simulink model "NeuralNetwork"  (R2016a)
settings: Solver=VariableStepAuto  StartTime=0.0  StopTime=100  RelTol=1e-3
values from neighbouring files (symbols this model uses):
  A0 = 0.5e-4    (= 5e-05)    [BPAndPID.m]
  cong = [1,1,1]/3600*d2r    [BPAndPID.m]
  fei1 = [5,5,5]'*d2r    [BPAndPID.m]
  HB0 = [IB*Wwo]'    [BPAndPID.m]
  invIB = inv(IB)    [BPAndPID.m]
  Noig = [1,1,1]*1/3*5*10^(-5)*d2r    [BPAndPID.m]
  Q0 = [Q1 Q2 Q3]    [BPAndPID.m]
  Q00 = 0.6736    [BPAndPID.m]
  Qt = [qt0 qt1 qt2 qt3]    [BPAndPID.m]
  Tscontrol = 0.05    [BPAndPID.m]
  Wc = [0 0 0]    [BPAndPID.m]
  Wio = [0 0.001 0]'    [BPAndPID.m]
libraries: aerolibutil x1
settings Model: Creator=lenovo  LastModifiedBy=lenovo

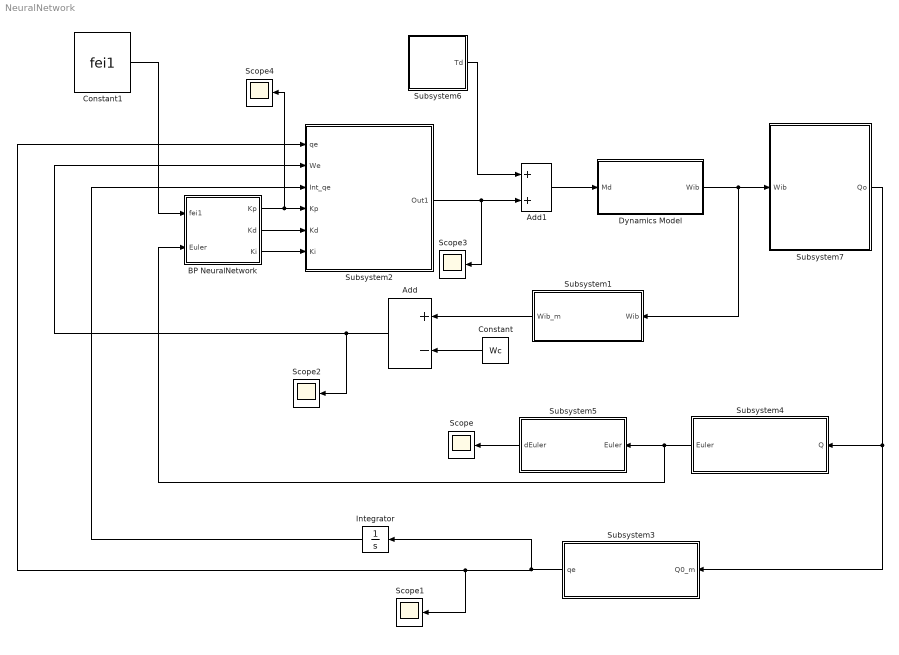
== system NeuralNetwork ==
  Add : Sum  Inputs=+-
  Add1 : Sum
  BP NeuralNetwork : Subsystem
  Constant : Constant  Value=Wc
  Constant1 : Constant  Value=fei1
  Dynamics Model : Subsystem
  Integrator : Integrator
  Scope{,1..4} (5 alike) : Scope
  Subsystem1 : Subsystem
      mask Display:
      | disp('Gyro')
      | port_label('input',1,'Wib')
      | port_label('output',1,'Wib_m')
  Subsystem2 : Subsystem
      mask Display:
      | disp('Controller')
      | port_label('input',1,'qe')
      | port_label('input',2,'we')
      | port_label('input',3,'int_qe')
      | port_label('input',4,'Kp')
      | port_label('input',5,'Kd')
      | port_label('input',6,'Ki')
      | port_label('output',1,'T')
  Subsystem3 : Subsystem
      mask Display:
      | disp('Target')
      | port_label('input',1,'Q')
      | port_label('output',1,'qe')
  Subsystem4 : Subsystem
      mask Display:
      | disp('Quaternion2Euler')
      | port_label('input',1,'Q')
      | port_label('output',1,'Euler')
  Subsystem5 : Subsystem
      mask Display:
      | disp('EulerError')
      | port_label('input',1,'Euler')
      | port_label('output',1,'dEuler')
  Subsystem6 : Subsystem
  Subsystem7 : Subsystem
      mask Display:
      | disp('Kinematics')
      | port_label('input',1,'Wib')
      | port_label('output',1,'Q')
  wires:
  Dynamics Model/1(Wib) -> Subsystem1/1(Wib), Subsystem7/1(Wib)
  Subsystem3/1(qe) -> Scope1/1, Subsystem2/1(qe), Integrator/1
  Subsystem7/1(Qo) -> Subsystem3/1(Q0_m), Subsystem4/1(Q)
  Subsystem5/1(dEuler) -> Scope/1
  Subsystem1/1(Wib_m) -> Add/1
  Constant/1 -> Add/2
  Add/1 -> Scope2/1, Subsystem2/2(We)
  Add1/1 -> Dynamics Model/1(Md)
  Subsystem2/1(Out1) -> Scope3/1, Add1/2
  Subsystem6/1(Td) -> Add1/1
  Integrator/1 -> Subsystem2/3(Int_qe)
  BP NeuralNetwork/1(Kp) -> Scope4/1, Subsystem2/4(Kp)
  BP NeuralNetwork/2(Kd) -> Subsystem2/5(Kd)
  BP NeuralNetwork/3(Ki) -> Subsystem2/6(Ki)
  Constant1/1 -> BP NeuralNetwork/1(fei1)
  Subsystem4/1(Euler) -> BP NeuralNetwork/2(Euler), Subsystem5/1(Euler)

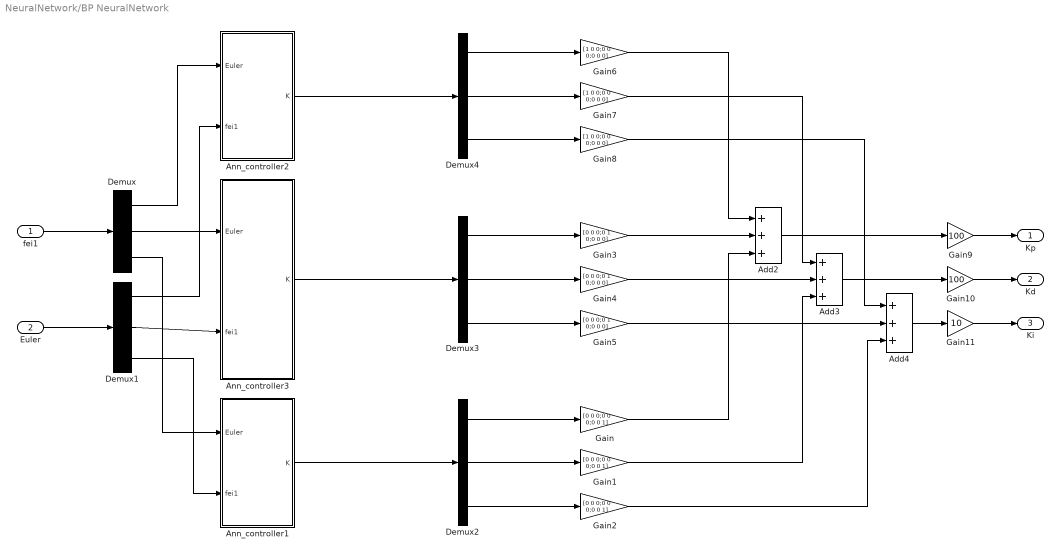
== system NeuralNetwork/BP NeuralNetwork ==
  fei1 : Inport
  Euler : Inport  Port=2
  Add2 : Sum  Inputs=+++
  Add3 : Sum  Inputs=+++
  Add4 : Sum  Inputs=+++
  Ann_controller1 : Subsystem
  Ann_controller2 : Subsystem
  Ann_controller3 : Subsystem
  Demux{,2..4} (4 alike) : Demux  Outputs=[1 1 1]
  Demux1 : Demux  Outputs=[1;1;1]
  Gain : Gain  Gain=[0 0 0;0 0 0;0 0 1]
  Gain1 : Gain  Gain=[0 0 0;0 0 0;0 0 1]
  Gain10 : Gain  Gain=100
  Gain11 : Gain  Gain=10
  Gain2 : Gain  Gain=[0 0 0;0 0 0;0 0 1]
  Gain3 : Gain  Gain=[0 0 0;0 1 0;0 0 0]
  Gain4 : Gain  Gain=[0 0 0;0 1 0;0 0 0]
  Gain5 : Gain  Gain=[0 0 0;0 1 0;0 0 0]
  Gain6 : Gain  Gain=[1 0 0;0 0 0;0 0 0]
  Gain7 : Gain  Gain=[1 0 0;0 0 0;0 0 0]
  Gain8 : Gain  Gain=[1 0 0;0 0 0;0 0 0]
  Gain9 : Gain  Gain=100
  Kp : Outport
  Kd : Outport  Port=2
  Ki : Outport  Port=3
  wires:
  Gain2/1 -> Add4/3
  Demux4/2 -> Gain7/1
  Demux2/3 -> Gain2/1
  Demux3/1 -> Gain3/1
  Gain6/1 -> Add2/1
  Gain3/1 -> Add2/2
  Demux2/2 -> Gain1/1
  Demux1/3 -> Ann_controller1/2(fei1)
  Demux3/2 -> Gain4/1
  Demux/1 -> Ann_controller2/1(Euler)
  Gain5/1 -> Add4/2
  Demux3/3 -> Gain5/1
  Demux2/1 -> Gain/1
  Demux4/3 -> Gain8/1
  Ann_controller2/1(K) -> Demux4/1
  Demux4/1 -> Gain6/1
  Gain/1 -> Add2/3
  Gain4/1 -> Add3/2
  Gain7/1 -> Add3/1
  Gain1/1 -> Add3/3
  Demux1/2 -> Ann_controller3/2(fei1)
  Demux1/1 -> Ann_controller2/2(fei1)
  Ann_controller3/1(K) -> Demux3/1
  Ann_controller1/1(K) -> Demux2/1
  Gain8/1 -> Add4/1
  Demux/2 -> Ann_controller3/1(Euler)
  fei1/1 -> Demux/1
  Euler/1 -> Demux1/1
  Add3/1 -> Gain10/1
  Add4/1 -> Gain11/1
  Add2/1 -> Gain9/1
  Gain9/1 -> Kp/1
  Gain10/1 -> Kd/1
  Gain11/1 -> Ki/1
  Demux/3 -> Ann_controller1/1(Euler)

== system NeuralNetwork/Dynamics Model ==
  note: W X H
  note: W
  note: H
  note: dH
  Md : Inport
  Add : Sum  Inputs=-+
  Gain : Gain  Gain=invIB  Multiplication=Matrix(u*K)
  Gain1 : Gain  Gain=-1
  Integrator : Integrator  InitialCondition=HB0
  Subsystem : Subsystem
      mask Display:
      | disp('Cross \nProduct')
      | port_label('input',1,'X')
      | port_label('input',2,'Y')
      | port_label('output',1,'X*Y')
  Wib : Outport
  wires:
  Integrator/1 -> Gain/1, Subsystem/2(Y)
  Gain/1 -> Wib/1, Gain1/1
  Add/1 -> Integrator/1
  Md/1 -> Add/2
  Gain1/1 -> Subsystem/1(X)
  Subsystem/1(X*Y) -> Add/1

== system NeuralNetwork/Subsystem1 ==
  Wib : Inport
  Add : Sum  Inputs=+++
  ConstantDrifting : Constant  Value=cong
  Gain : Gain  Gain=Noig
  Quantizer : Quantizer  QuantizationInterval=Gyquan
  WhiteNoise : RandomNumber  Mean=[0,0,0]  Variance=[1,1,1]  Seed=fix(abs(10000*rand([3,1])))  SampleTime=Tscontrol
  Wib_m : Outport
  wires:
  Quantizer/1 -> Wib_m/1
  Wib/1 -> Add/2
  Add/1 -> Quantizer/1
  ConstantDrifting/1 -> Add/3
  Gain/1 -> Add/1
  WhiteNoise/1 -> Gain/1

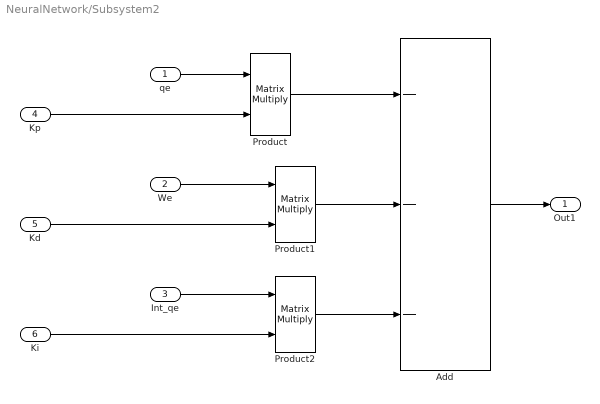
== system NeuralNetwork/Subsystem2 ==
  qe : Inport
  We : Inport  Port=2
  Int_qe : Inport  Port=3
  Kp : Inport  Port=4
  Kd : Inport  Port=5
  Ki : Inport  Port=6
  Add : Sum  Inputs=---
  Product : Product  Multiplication=Matrix(*)
  Product1 : Product  Multiplication=Matrix(*)
  Product2 : Product  Multiplication=Matrix(*)
  Out1 : Outport
  wires:
  Add/1 -> Out1/1
  Product/1 -> Add/1
  Kd/1 -> Product1/2
  We/1 -> Product1/1
  Product1/1 -> Add/2
  Kp/1 -> Product/2
  qe/1 -> Product/1
  Product2/1 -> Add/3
  Ki/1 -> Product2/2
  Int_qe/1 -> Product2/1

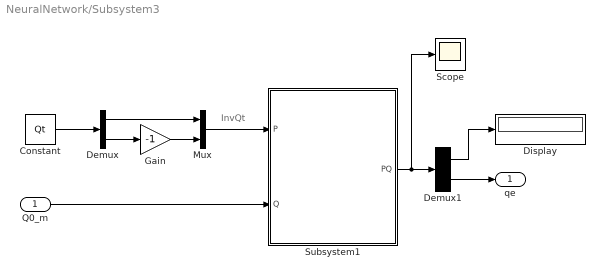
== system NeuralNetwork/Subsystem3 ==
  note: InvQt
  Q0_m : Inport
  Constant : Constant  Value=Qt
  Demux : Demux  Outputs=2
  Demux1 : Demux  Outputs=[1 3]
  Display : Display
  Gain : Gain  Gain=-1
  Mux : Mux  Inputs=2
  Scope : Scope
  Subsystem1 : Subsystem
      mask Display:
      | disp('InterQ Multiply')
      | port_label('input',1,'P')
      | port_label('input',2,'Q')
      | port_label('output',1,'PQ')
  qe : Outport
  wires:
  Subsystem1/1(PQ) -> Scope/1, Demux1/1
  Constant/1 -> Demux/1
  Demux/1 -> Mux/1
  Demux/2 -> Gain/1
  Gain/1 -> Mux/2
  Q0_m/1 -> Subsystem1/2(Q)
  Mux/1 -> Subsystem1/1(P)
  Demux1/2 -> qe/1
  Demux1/1 -> Display/1

== system NeuralNetwork/Subsystem4 ==
  Q : Inport
  Mux : Mux  Inputs=3
  Phi : Fcn  Expr=atan(2*(u(1)*u(4)-u(3)*u(2))/(2*(u(1)^2+u(3)^2)-1))
  Psi : Fcn  Expr=atan(2*(u(1)*u(3)-u(2)*u(4))/(2*(u(1)^2+u(4)^2)-1))
  Scope : Scope
  Theta : Fcn  Expr=asin(2*(u(1)*u(2)+u(4)*u(3)))
  Euler : Outport
  wires:
  Mux/1 -> Scope/1, Euler/1
  Q/1 -> Theta/1, Phi/1, Psi/1
  Theta/1 -> Mux/3
  Psi/1 -> Mux/1
  Phi/1 -> Mux/2

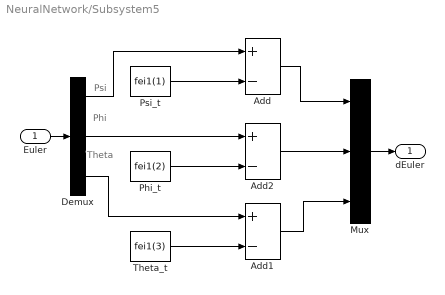
== system NeuralNetwork/Subsystem5 ==
  note: Psi
  note: Theta
  note: Phi
  Euler : Inport
  Add : Sum  Inputs=+-
  Add1 : Sum  Inputs=+-
  Add2 : Sum  Inputs=+-
  Demux : Demux  Outputs=[1 1 1]
  Mux : Mux  Inputs=3
  Phi_t : Constant  Value=fei1(2)
  Psi_t : Constant  Value=fei1(1)
  Theta_t : Constant  Value=fei1(3)
  dEuler : Outport
  wires:
  Demux/1 -> Add/1
  Mux/1 -> dEuler/1
  Euler/1 -> Demux/1
  Theta_t/1 -> Add1/2
  Add/1 -> Mux/1
  Demux/3 -> Add1/1
  Add2/1 -> Mux/2
  Psi_t/1 -> Add/2
  Demux/2 -> Add2/1
  Phi_t/1 -> Add2/2
  Add1/1 -> Mux/3

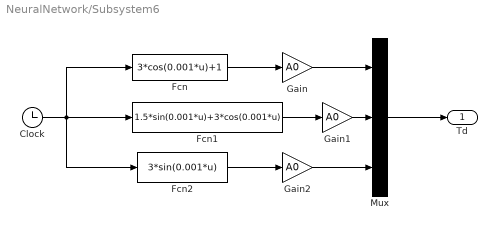
== system NeuralNetwork/Subsystem6 ==
  Clock : Clock
  Fcn : Fcn  Expr=3*cos(0.001*u)+1
  Fcn1 : Fcn  Expr=1.5*sin(0.001*u)+3*cos(0.001*u)
  Fcn2 : Fcn  Expr=3*sin(0.001*u)
  Gain : Gain  Gain=A0
  Gain1 : Gain  Gain=A0
  Gain2 : Gain  Gain=A0
  Mux : Mux  Inputs=3
  Td : Outport
  wires:
  Gain/1 -> Mux/1
  Mux/1 -> Td/1
  Clock/1 -> Fcn2/1, Fcn/1, Fcn1/1
  Fcn2/1 -> Gain2/1
  Fcn1/1 -> Gain1/1
  Fcn/1 -> Gain/1
  Gain2/1 -> Mux/3
  Gain1/1 -> Mux/2

== system NeuralNetwork/Subsystem7 ==
  Wib : Inport
  Add1 : Sum  Inputs=+-
  Constant : Constant  Value=Wio
  Product1 : Product  Multiplication=Matrix(*)
  Subsystem1 : Subsystem
      mask Display:
      | disp('Quaternion2 \nAttitudeMarix')
      | port_label('input',1,'Qua')
      | port_label('output',1,'Marix')
  Subsystem5 : Subsystem
      mask Display:
      | disp('Quaternion \nSolve Model')
      | port_label('input',1,'Wob')
      | port_label('output',1,'Qo')
  Qo : Outport
  wires:
  Subsystem5/1(Out1) -> Qo/1, Subsystem1/1(Quaternion)
  Constant/1 -> Product1/2
  Subsystem1/1("AttitudeMarix ") -> Product1/1
  Add1/1 -> Subsystem5/1(In1)
  Wib/1 -> Add1/1
  Product1/1 -> Add1/2

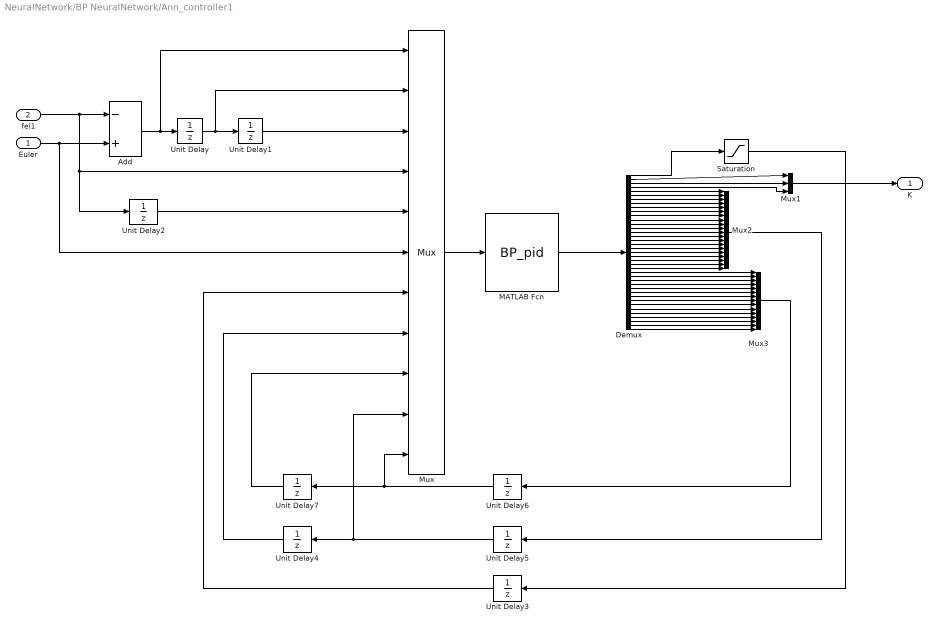
== system NeuralNetwork/BP NeuralNetwork/Ann_controller1 ==
  Euler : Inport
  fei1 : Inport  Port=2
  Add : Sum  Inputs=-+
  Demux : Demux  Outputs=39
  MATLAB Fcn : MATLABFcn  MATLABFcn=BP_pid  Output1D=off
  Mux : Mux  Inputs=11
  Mux1 : Mux  Inputs=3
  Mux2 : Mux  Inputs=20
  Mux3 : Mux  Inputs=15
  Saturation : Saturate  UpperLimit=1  LowerLimit=0
  Unit Delay{,1..3} (4 alike) : UnitDelay
  Unit Delay4 : UnitDelay  InitialCondition=rand(20,1)
  Unit Delay5 : UnitDelay  InitialCondition=rand(20,1)
  Unit Delay6 : UnitDelay  InitialCondition=rand(15,1)
  Unit Delay7 : UnitDelay  InitialCondition=rand(15,1)
  K : Outport
  wires:
  Euler/1 -> Mux/6, Add/2
  Add/1 -> Mux/1, Unit Delay/1
  Unit Delay/1 -> Mux/2, Unit Delay1/1
  MATLAB Fcn/1 -> Demux/1
  Unit Delay5/1 -> Unit Delay4/1, Mux/10
  Unit Delay3/1 -> Mux/7
  Unit Delay6/1 -> Unit Delay7/1, Mux/11
  Demux/2 -> Mux1/1
  Demux/3 -> Mux1/2
  Demux/4 -> Mux1/3
  Mux1/1 -> K/1
  Demux/5 -> Mux2/1
  Demux/6 -> Mux2/2
  Demux/7 -> Mux2/3
  Demux/8 -> Mux2/4
  Demux/9 -> Mux2/5
  Demux/10 -> Mux2/6
  Demux/11 -> Mux2/7
  Demux/12 -> Mux2/8
  Demux/13 -> Mux2/9
  Demux/14 -> Mux2/10
  Demux/15 -> Mux2/11
  Demux/16 -> Mux2/12
  Demux/17 -> Mux2/13
  Demux/18 -> Mux2/14
  Demux/19 -> Mux2/15
  Demux/20 -> Mux2/16
  Demux/21 -> Mux2/17
  Demux/22 -> Mux2/18
  Demux/23 -> Mux2/19
  Demux/24 -> Mux2/20
  Mux2/1 -> Unit Delay5/1
  Demux/25 -> Mux3/1
  Demux/26 -> Mux3/2
  Demux/27 -> Mux3/3
  Demux/28 -> Mux3/4
  Demux/29 -> Mux3/5
  Demux/30 -> Mux3/6
  Demux/31 -> Mux3/7
  Demux/32 -> Mux3/8
  Demux/33 -> Mux3/9
  Demux/34 -> Mux3/10
  Demux/35 -> Mux3/11
  Demux/36 -> Mux3/12
  Demux/37 -> Mux3/13
  Demux/38 -> Mux3/14
  Demux/39 -> Mux3/15
  Mux3/1 -> Unit Delay6/1
  Demux/1 -> Saturation/1
  Saturation/1 -> Unit Delay3/1
  Mux/1 -> MATLAB Fcn/1
  Unit Delay7/1 -> Mux/9
  Unit Delay4/1 -> Mux/8
  fei1/1 -> Unit Delay2/1, Mux/4, Add/1
  Unit Delay2/1 -> Mux/5
  Unit Delay1/1 -> Mux/3

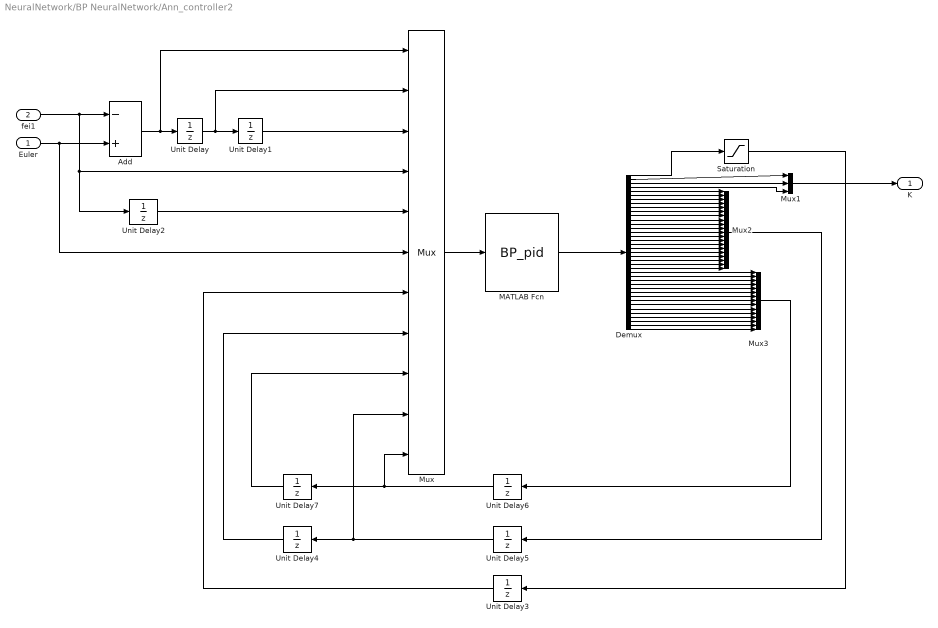
== system NeuralNetwork/BP NeuralNetwork/Ann_controller2 ==
  Euler : Inport
  fei1 : Inport  Port=2
  Add : Sum  Inputs=-+
  Demux : Demux  Outputs=39
  MATLAB Fcn : MATLABFcn  MATLABFcn=BP_pid  Output1D=off
  Mux : Mux  Inputs=11
  Mux1 : Mux  Inputs=3
  Mux2 : Mux  Inputs=20
  Mux3 : Mux  Inputs=15
  Saturation : Saturate  UpperLimit=1  LowerLimit=0
  Unit Delay{,1..3} (4 alike) : UnitDelay
  Unit Delay4 : UnitDelay  InitialCondition=rand(20,1)
  Unit Delay5 : UnitDelay  InitialCondition=rand(20,1)
  Unit Delay6 : UnitDelay  InitialCondition=rand(15,1)
  Unit Delay7 : UnitDelay  InitialCondition=rand(15,1)
  K : Outport
  wires:
  Euler/1 -> Mux/6, Add/2
  Add/1 -> Mux/1, Unit Delay/1
  Unit Delay/1 -> Mux/2, Unit Delay1/1
  MATLAB Fcn/1 -> Demux/1
  Unit Delay5/1 -> Unit Delay4/1, Mux/10
  Unit Delay3/1 -> Mux/7
  Unit Delay6/1 -> Unit Delay7/1, Mux/11
  Demux/2 -> Mux1/1
  Demux/3 -> Mux1/2
  Demux/4 -> Mux1/3
  Mux1/1 -> K/1
  Demux/5 -> Mux2/1
  Demux/6 -> Mux2/2
  Demux/7 -> Mux2/3
  Demux/8 -> Mux2/4
  Demux/9 -> Mux2/5
  Demux/10 -> Mux2/6
  Demux/11 -> Mux2/7
  Demux/12 -> Mux2/8
  Demux/13 -> Mux2/9
  Demux/14 -> Mux2/10
  Demux/15 -> Mux2/11
  Demux/16 -> Mux2/12
  Demux/17 -> Mux2/13
  Demux/18 -> Mux2/14
  Demux/19 -> Mux2/15
  Demux/20 -> Mux2/16
  Demux/21 -> Mux2/17
  Demux/22 -> Mux2/18
  Demux/23 -> Mux2/19
  Demux/24 -> Mux2/20
  Mux2/1 -> Unit Delay5/1
  Demux/25 -> Mux3/1
  Demux/26 -> Mux3/2
  Demux/27 -> Mux3/3
  Demux/28 -> Mux3/4
  Demux/29 -> Mux3/5
  Demux/30 -> Mux3/6
  Demux/31 -> Mux3/7
  Demux/32 -> Mux3/8
  Demux/33 -> Mux3/9
  Demux/34 -> Mux3/10
  Demux/35 -> Mux3/11
  Demux/36 -> Mux3/12
  Demux/37 -> Mux3/13
  Demux/38 -> Mux3/14
  Demux/39 -> Mux3/15
  Mux3/1 -> Unit Delay6/1
  Demux/1 -> Saturation/1
  Saturation/1 -> Unit Delay3/1
  Mux/1 -> MATLAB Fcn/1
  Unit Delay7/1 -> Mux/9
  Unit Delay4/1 -> Mux/8
  fei1/1 -> Unit Delay2/1, Mux/4, Add/1
  Unit Delay2/1 -> Mux/5
  Unit Delay1/1 -> Mux/3

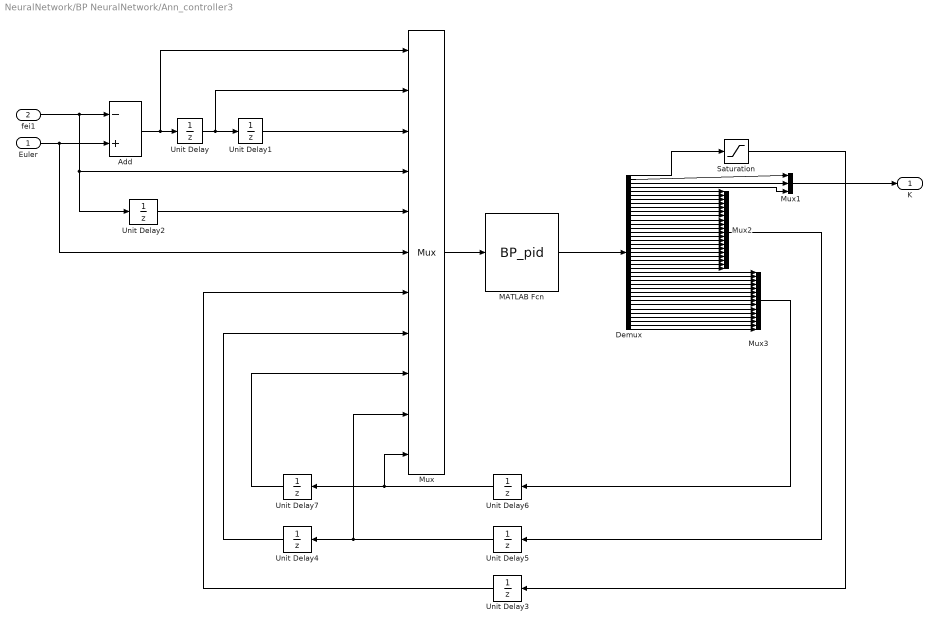
== system NeuralNetwork/BP NeuralNetwork/Ann_controller3 ==
  Euler : Inport
  fei1 : Inport  Port=2
  Add : Sum  Inputs=-+
  Demux : Demux  Outputs=39
  MATLAB Fcn : MATLABFcn  MATLABFcn=BP_pid  Output1D=off
  Mux : Mux  Inputs=11
  Mux1 : Mux  Inputs=3
  Mux2 : Mux  Inputs=20
  Mux3 : Mux  Inputs=15
  Saturation : Saturate  UpperLimit=1  LowerLimit=0
  Unit Delay{,1..3} (4 alike) : UnitDelay
  Unit Delay4 : UnitDelay  InitialCondition=rand(20,1)
  Unit Delay5 : UnitDelay  InitialCondition=rand(20,1)
  Unit Delay6 : UnitDelay  InitialCondition=rand(15,1)
  Unit Delay7 : UnitDelay  InitialCondition=rand(15,1)
  K : Outport
  wires:
  Euler/1 -> Mux/6, Add/2
  Add/1 -> Mux/1, Unit Delay/1
  Unit Delay/1 -> Mux/2, Unit Delay1/1
  MATLAB Fcn/1 -> Demux/1
  Unit Delay5/1 -> Unit Delay4/1, Mux/10
  Unit Delay3/1 -> Mux/7
  Unit Delay6/1 -> Unit Delay7/1, Mux/11
  Demux/2 -> Mux1/1
  Demux/3 -> Mux1/2
  Demux/4 -> Mux1/3
  Mux1/1 -> K/1
  Demux/5 -> Mux2/1
  Demux/6 -> Mux2/2
  Demux/7 -> Mux2/3
  Demux/8 -> Mux2/4
  Demux/9 -> Mux2/5
  Demux/10 -> Mux2/6
  Demux/11 -> Mux2/7
  Demux/12 -> Mux2/8
  Demux/13 -> Mux2/9
  Demux/14 -> Mux2/10
  Demux/15 -> Mux2/11
  Demux/16 -> Mux2/12
  Demux/17 -> Mux2/13
  Demux/18 -> Mux2/14
  Demux/19 -> Mux2/15
  Demux/20 -> Mux2/16
  Demux/21 -> Mux2/17
  Demux/22 -> Mux2/18
  Demux/23 -> Mux2/19
  Demux/24 -> Mux2/20
  Mux2/1 -> Unit Delay5/1
  Demux/25 -> Mux3/1
  Demux/26 -> Mux3/2
  Demux/27 -> Mux3/3
  Demux/28 -> Mux3/4
  Demux/29 -> Mux3/5
  Demux/30 -> Mux3/6
  Demux/31 -> Mux3/7
  Demux/32 -> Mux3/8
  Demux/33 -> Mux3/9
  Demux/34 -> Mux3/10
  Demux/35 -> Mux3/11
  Demux/36 -> Mux3/12
  Demux/37 -> Mux3/13
  Demux/38 -> Mux3/14
  Demux/39 -> Mux3/15
  Mux3/1 -> Unit Delay6/1
  Demux/1 -> Saturation/1
  Saturation/1 -> Unit Delay3/1
  Mux/1 -> MATLAB Fcn/1
  Unit Delay7/1 -> Mux/9
  Unit Delay4/1 -> Mux/8
  fei1/1 -> Unit Delay2/1, Mux/4, Add/1
  Unit Delay2/1 -> Mux/5
  Unit Delay1/1 -> Mux/3

== system NeuralNetwork/Dynamics Model/Subsystem ==
  X : Inport
  Y : Inport  Port=2
  Fcn : Fcn  Expr=u[2]*u[6]-u[3]*u[5]
  Fcn1 : Fcn  Expr=u[3]*u[4]-u[1]*u[6]
  Fcn2 : Fcn  Expr=u[1]*u[5]-u[2]*u[4]
  Mux : Mux  Inputs=[1 1 1]
  Mux1 : Mux  Inputs=[3 3]
  X*Y : Outport
  wires:
  X/1 -> Mux1/1
  Y/1 -> Mux1/2
  Mux1/1 -> Fcn2/1, Fcn1/1, Fcn/1
  Fcn/1 -> Mux/1
  Mux/1 -> X*Y/1
  Fcn1/1 -> Mux/2
  Fcn2/1 -> Mux/3

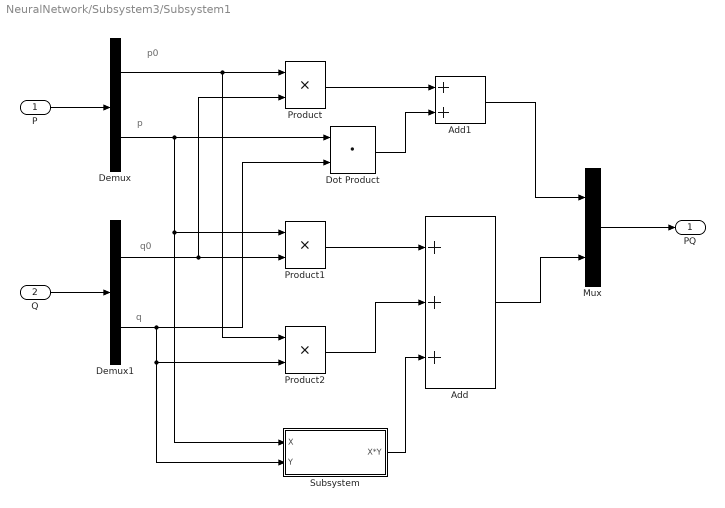
== system NeuralNetwork/Subsystem3/Subsystem1 ==
  note: q
  note: q0
  note: p
  note: p0
  P : Inport
  Q : Inport  Port=2
  Add : Sum  Inputs=+++
  Add1 : Sum
  Demux : Demux  Outputs=[1 3]
  Demux1 : Demux  Outputs=[1 3]
  Dot Product : DotProduct  InputSameDT=on  OutDataTypeStr=Inherit: Inherit via internal rule
  Mux : Mux  Inputs=2
  Product : Product
  Product1 : Product
  Product2 : Product
  Subsystem : Subsystem
      mask Display:
      | disp('Cross \nProduct')
      | port_label('input',1,'X')
      | port_label('input',2,'Y')
      | port_label('output',1,'X*Y')
  PQ : Outport
  wires:
  P/1 -> Demux/1
  Q/1 -> Demux1/1
  Demux/1 -> Product2/1, Product/1
  Demux/2 -> Product1/1, Subsystem/1(X), Dot Product/1
  Demux1/1 -> Product/2, Product1/2
  Demux1/2 -> Product2/2, Subsystem/2(Y), Dot Product/2
  Product/1 -> Add1/1
  Dot Product/1 -> Add1/2
  Product1/1 -> Add/1
  Product2/1 -> Add/2
  Subsystem/1(X*Y) -> Add/3
  Add1/1 -> Mux/1
  Add/1 -> Mux/2
  Mux/1 -> PQ/1

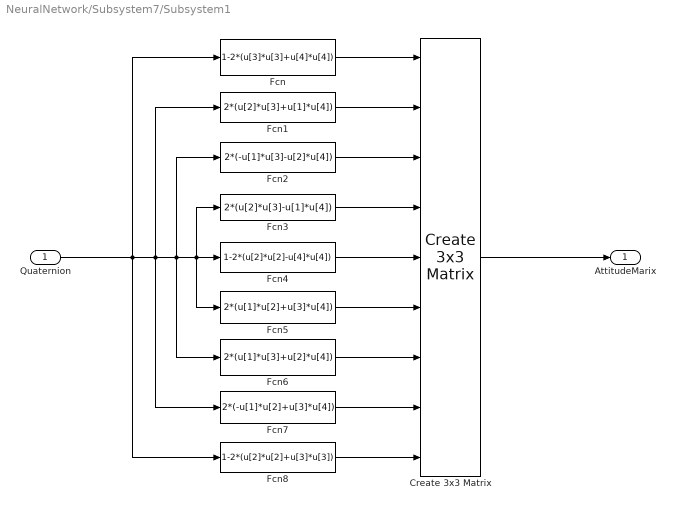
== system NeuralNetwork/Subsystem7/Subsystem1 ==
  Quaternion : Inport
  Create 3x3 Matrix : aerolibutil/Create 3x3 Matrix
  Fcn : Fcn  Expr=1-2*(u[3]*u[3]+u[4]*u[4])
  Fcn1 : Fcn  Expr=2*(u[2]*u[3]+u[1]*u[4])
  Fcn2 : Fcn  Expr=2*(-u[1]*u[3]-u[2]*u[4])
  Fcn3 : Fcn  Expr=2*(u[2]*u[3]-u[1]*u[4])
  Fcn4 : Fcn  Expr=1-2*(u[2]*u[2]-u[4]*u[4])
  Fcn5 : Fcn  Expr=2*(u[1]*u[2]+u[3]*u[4])
  Fcn6 : Fcn  Expr=2*(u[1]*u[3]+u[2]*u[4])
  Fcn7 : Fcn  Expr=2*(-u[1]*u[2]+u[3]*u[4])
  Fcn8 : Fcn  Expr=1-2*(u[2]*u[2]+u[3]*u[3])
  "AttitudeMarix " : Outport
  wires:
  Fcn6/1 -> Create 3x3 Matrix/7
  Quaternion/1 -> Fcn8/1, Fcn/1, Fcn7/1, Fcn6/1, Fcn2/1, Fcn5/1, Fcn3/1, Fcn4/1, Fcn1/1
  Create 3x3 Matrix/1 -> "AttitudeMarix "/1
  Fcn/1 -> Create 3x3 Matrix/1
  Fcn1/1 -> Create 3x3 Matrix/2
  Fcn2/1 -> Create 3x3 Matrix/3
  Fcn3/1 -> Create 3x3 Matrix/4
  Fcn4/1 -> Create 3x3 Matrix/5
  Fcn5/1 -> Create 3x3 Matrix/6
  Fcn7/1 -> Create 3x3 Matrix/8
  Fcn8/1 -> Create 3x3 Matrix/9

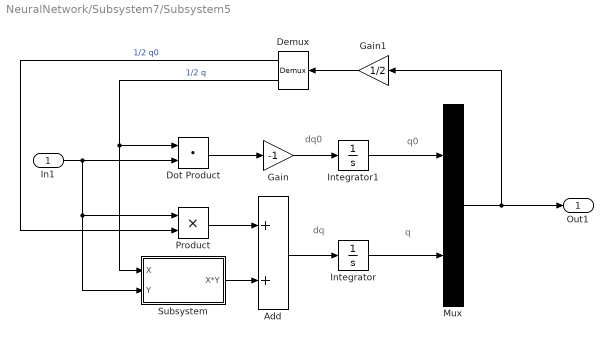
== system NeuralNetwork/Subsystem7/Subsystem5 ==
  note: q
  note: dq
  note: q0
  note: dq0
  In1 : Inport
  Add : Sum
  Demux : Demux  Outputs=[1 3]
  Dot Product : DotProduct  InputSameDT=on  OutDataTypeStr=Inherit: Inherit via internal rule
  Gain : Gain  Gain=-1
  Gain1 : Gain  Gain=1/2
  Integrator : Integrator  InitialCondition=Q0
  Integrator1 : Integrator  InitialCondition=Q00
  Mux : Mux  Inputs=2
  Product : Product
  Subsystem : Subsystem
      mask Display:
      | disp('Cross \nProduct')
      | port_label('input',1,'X')
      | port_label('input',2,'Y')
      | port_label('output',1,'X*Y')
  Out1 : Outport
  wires:
  Gain/1 -> Integrator1/1
  Add/1 -> Integrator/1
  Mux/1 -> Gain1/1, Out1/1
  Integrator1/1 -> Mux/1
  Integrator/1 -> Mux/2
  Gain1/1 -> Demux/1
  In1/1 -> Product/1, Subsystem/2(Y), Dot Product/2
  Dot Product/1 -> Gain/1
  Demux/2 -> Dot Product/1, Subsystem/1(X)  "1/2 q"
  Product/1 -> Add/1
  Demux/1 -> Product/2  "1/2 q0"
  Subsystem/1(X*Y) -> Add/2

== system NeuralNetwork/Subsystem3/Subsystem1/Subsystem ==
  X : Inport
  Y : Inport  Port=2
  Fcn : Fcn  Expr=u[2]*u[6]-u[3]*u[5]
  Fcn1 : Fcn  Expr=u[3]*u[4]-u[1]*u[6]
  Fcn2 : Fcn  Expr=u[1]*u[5]-u[2]*u[4]
  Mux : Mux  Inputs=[1 1 1]
  Mux1 : Mux  Inputs=[3 3]
  X*Y : Outport
  wires:
  X/1 -> Mux1/1
  Y/1 -> Mux1/2
  Mux1/1 -> Fcn2/1, Fcn1/1, Fcn/1
  Fcn/1 -> Mux/1
  Mux/1 -> X*Y/1
  Fcn1/1 -> Mux/2
  Fcn2/1 -> Mux/3

== system NeuralNetwork/Subsystem7/Subsystem5/Subsystem ==
  X : Inport
  Y : Inport  Port=2
  Fcn : Fcn  Expr=u[2]*u[6]-u[3]*u[5]
  Fcn1 : Fcn  Expr=u[3]*u[4]-u[1]*u[6]
  Fcn2 : Fcn  Expr=u[1]*u[5]-u[2]*u[4]
  Mux : Mux  Inputs=[1 1 1]
  Mux1 : Mux  Inputs=[3 3]
  X*Y : Outport
  wires:
  X/1 -> Mux1/1
  Y/1 -> Mux1/2
  Mux1/1 -> Fcn2/1, Fcn1/1, Fcn/1
  Fcn/1 -> Mux/1
  Mux/1 -> X*Y/1
  Fcn1/1 -> Mux/2
  Fcn2/1 -> Mux/3
